simulink model "SIM_PEM_stack"  (R2020b)
settings: Solver=VariableStepAuto  StartTime=0.0  StopTime=60e3  RelTol=1e-3
undefined symbols (not defined in the file or in its folder): FC, FuelCellLoadFcn, gcbh, sps_rtmsupport
libraries: powerlib x106, simulink x22, spsFuelCellModel x21, dspswit3 x1, mylib x1
(part 3 of 3)

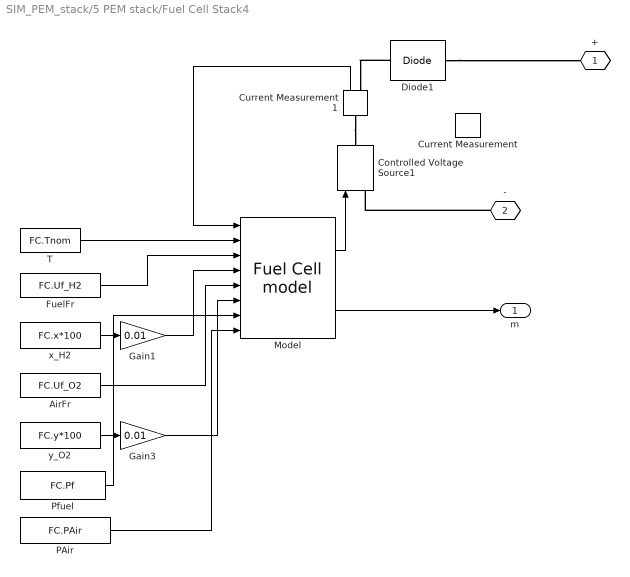
== system SIM_PEM_stack/5 PEM stack/Fuel Cell Stack4 ==
  AirFr : Constant  Value=FC.Uf_O2
  Controlled Voltage Source1 : powerlib/Electrical Sources/Controlled Voltage Source  Initialize=on  Source_Type=AC  Amplitude=0  Phase=0  Frequency=0  Measurements=None
  Current Measurement : powerlib/Measurements/Current Measurement  PhasorSimulation=off  OutputType=Complex  PSBequivalent=0
  Current Measurement1 : powerlib/Measurements/Current Measurement  PhasorSimulation=off  OutputType=Complex  PSBequivalent=0
  Diode1 : powerlib/Power Electronics/Diode  Ron=FC.Rohm  Lon=0  Vf=0  IC=0  UseSnubber=off  Rs=1e4  Cs=inf  Measurements=off
  FuelFr : Constant  Value=FC.Uf_H2
  Gain1 : Gain  Gain=0.01
  Gain3 : Gain  Gain=0.01
  Model : spsFuelCellModel/Fuel Cell model  SystemSampleTime=-1  LabelModeActiveChoice=Continuous/Detailed  VariantActivationTime=update diagram  Latency=0  AutoFrameSizeCalculation=off
      settings: AttributesFormatString=%<BlockChoice>  SourceProductBaseCode=PS
  PAir : Constant  Value=FC.PAir
  Pfuel : Constant  Value=FC.Pf
  T : Constant  Value=FC.Tnom
  x_H2 : Constant  Value=FC.x*100
  y_O2 : Constant  Value=FC.y*100
  + : PMIOPort  Tag=PMCPort  Side=Right
  - : PMIOPort  Tag=PMCPort  Port=2  Side=Right
  m : Outport  VectorParamsAs1DForOutWhenUnconnected=off
  wires:
  PAir/1 -> Model/8
  Pfuel/1 -> Model/7
  T/1 -> Model/2
  Model/1 -> Controlled Voltage Source1/1
  Current Measurement1/1 -> Model/1
  Model/2 -> m/1
  FuelFr/1 -> Model/3
  x_H2/1 -> Gain1/1
  AirFr/1 -> Model/5
  y_O2/1 -> Gain3/1
  Gain1/1 -> Model/4
  Gain3/1 -> Model/6
  connections:
  Current Measurement1/LConn1 -- Controlled Voltage Source1/RConn1
  Diode1/LConn1 -- Current Measurement1/RConn1
  -/RConn1 -- Controlled Voltage Source1/LConn1
  Diode1/RConn1 -- +/RConn1

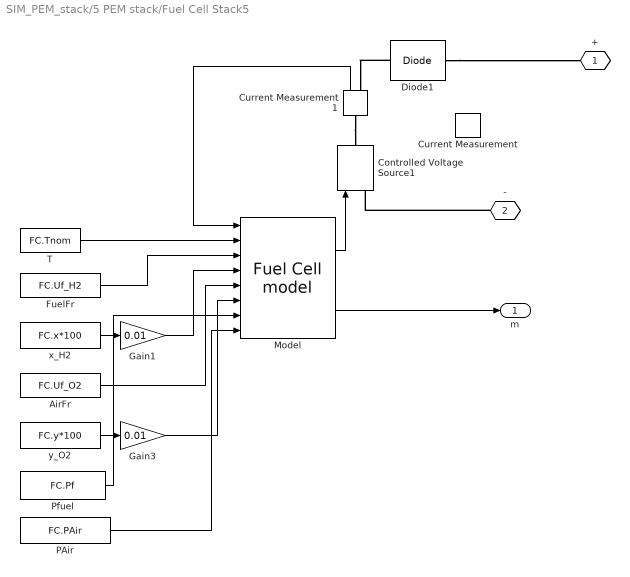
== system SIM_PEM_stack/5 PEM stack/Fuel Cell Stack5 ==
  AirFr : Constant  Value=FC.Uf_O2
  Controlled Voltage Source1 : powerlib/Electrical Sources/Controlled Voltage Source  Initialize=on  Source_Type=AC  Amplitude=0  Phase=0  Frequency=0  Measurements=None
  Current Measurement : powerlib/Measurements/Current Measurement  PhasorSimulation=off  OutputType=Complex  PSBequivalent=0
  Current Measurement1 : powerlib/Measurements/Current Measurement  PhasorSimulation=off  OutputType=Complex  PSBequivalent=0
  Diode1 : powerlib/Power Electronics/Diode  Ron=FC.Rohm  Lon=0  Vf=0  IC=0  UseSnubber=off  Rs=1e4  Cs=inf  Measurements=off
  FuelFr : Constant  Value=FC.Uf_H2
  Gain1 : Gain  Gain=0.01
  Gain3 : Gain  Gain=0.01
  Model : spsFuelCellModel/Fuel Cell model  SystemSampleTime=-1  LabelModeActiveChoice=Continuous/Detailed  VariantActivationTime=update diagram  Latency=0  AutoFrameSizeCalculation=off
      settings: AttributesFormatString=%<BlockChoice>  SourceProductBaseCode=PS
  PAir : Constant  Value=FC.PAir
  Pfuel : Constant  Value=FC.Pf
  T : Constant  Value=FC.Tnom
  x_H2 : Constant  Value=FC.x*100
  y_O2 : Constant  Value=FC.y*100
  + : PMIOPort  Tag=PMCPort  Side=Right
  - : PMIOPort  Tag=PMCPort  Port=2  Side=Right
  m : Outport  VectorParamsAs1DForOutWhenUnconnected=off
  wires:
  PAir/1 -> Model/8
  Pfuel/1 -> Model/7
  T/1 -> Model/2
  Model/1 -> Controlled Voltage Source1/1
  Current Measurement1/1 -> Model/1
  Model/2 -> m/1
  FuelFr/1 -> Model/3
  x_H2/1 -> Gain1/1
  AirFr/1 -> Model/5
  y_O2/1 -> Gain3/1
  Gain1/1 -> Model/4
  Gain3/1 -> Model/6
  connections:
  Current Measurement1/LConn1 -- Controlled Voltage Source1/RConn1
  Diode1/LConn1 -- Current Measurement1/RConn1
  -/RConn1 -- Controlled Voltage Source1/LConn1
  Diode1/RConn1 -- +/RConn1

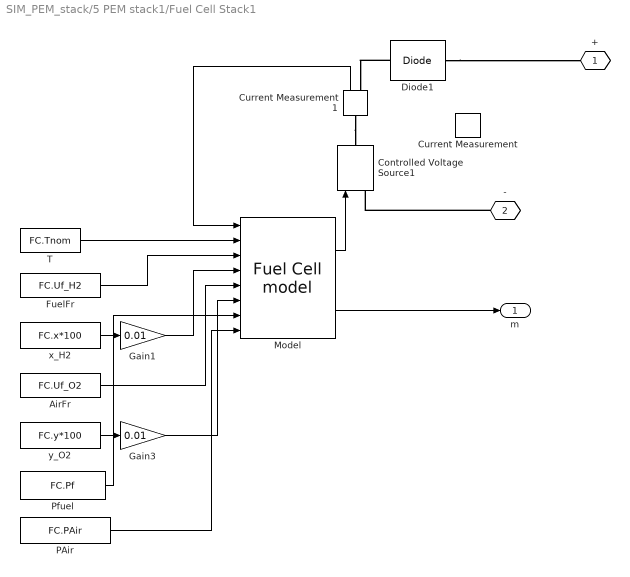
== system SIM_PEM_stack/5 PEM stack1/Fuel Cell Stack1 ==
  AirFr : Constant  Value=FC.Uf_O2
  Controlled Voltage Source1 : powerlib/Electrical Sources/Controlled Voltage Source  Initialize=on  Source_Type=AC  Amplitude=0  Phase=0  Frequency=0  Measurements=None
  Current Measurement : powerlib/Measurements/Current Measurement  PhasorSimulation=off  OutputType=Complex  PSBequivalent=0
  Current Measurement1 : powerlib/Measurements/Current Measurement  PhasorSimulation=off  OutputType=Complex  PSBequivalent=0
  Diode1 : powerlib/Power Electronics/Diode  Ron=FC.Rohm  Lon=0  Vf=0  IC=0  UseSnubber=off  Rs=1e4  Cs=inf  Measurements=off
  FuelFr : Constant  Value=FC.Uf_H2
  Gain1 : Gain  Gain=0.01
  Gain3 : Gain  Gain=0.01
  Model : spsFuelCellModel/Fuel Cell model  SystemSampleTime=-1  LabelModeActiveChoice=Continuous/Detailed  VariantActivationTime=update diagram  Latency=0  AutoFrameSizeCalculation=off
      settings: AttributesFormatString=%<BlockChoice>  SourceProductBaseCode=PS
  PAir : Constant  Value=FC.PAir
  Pfuel : Constant  Value=FC.Pf
  T : Constant  Value=FC.Tnom
  x_H2 : Constant  Value=FC.x*100
  y_O2 : Constant  Value=FC.y*100
  + : PMIOPort  Tag=PMCPort  Side=Right
  - : PMIOPort  Tag=PMCPort  Port=2  Side=Right
  m : Outport  VectorParamsAs1DForOutWhenUnconnected=off
  wires:
  PAir/1 -> Model/8
  Pfuel/1 -> Model/7
  T/1 -> Model/2
  Model/1 -> Controlled Voltage Source1/1
  Current Measurement1/1 -> Model/1
  Model/2 -> m/1
  FuelFr/1 -> Model/3
  x_H2/1 -> Gain1/1
  AirFr/1 -> Model/5
  y_O2/1 -> Gain3/1
  Gain1/1 -> Model/4
  Gain3/1 -> Model/6
  connections:
  Current Measurement1/LConn1 -- Controlled Voltage Source1/RConn1
  Diode1/LConn1 -- Current Measurement1/RConn1
  -/RConn1 -- Controlled Voltage Source1/LConn1
  Diode1/RConn1 -- +/RConn1

== system SIM_PEM_stack/5 PEM stack1/Fuel Cell Stack2 ==
  AirFr : Constant  Value=FC.Uf_O2
  Controlled Voltage Source1 : powerlib/Electrical Sources/Controlled Voltage Source  Initialize=on  Source_Type=AC  Amplitude=0  Phase=0  Frequency=0  Measurements=None
  Current Measurement : powerlib/Measurements/Current Measurement  PhasorSimulation=off  OutputType=Complex  PSBequivalent=0
  Current Measurement1 : powerlib/Measurements/Current Measurement  PhasorSimulation=off  OutputType=Complex  PSBequivalent=0
  Diode1 : powerlib/Power Electronics/Diode  Ron=FC.Rohm  Lon=0  Vf=0  IC=0  UseSnubber=off  Rs=1e4  Cs=inf  Measurements=off
  FuelFr : Constant  Value=FC.Uf_H2
  Gain1 : Gain  Gain=0.01
  Gain3 : Gain  Gain=0.01
  Model : spsFuelCellModel/Fuel Cell model  SystemSampleTime=-1  LabelModeActiveChoice=Continuous/Detailed  VariantActivationTime=update diagram  Latency=0  AutoFrameSizeCalculation=off
      settings: AttributesFormatString=%<BlockChoice>  SourceProductBaseCode=PS
  PAir : Constant  Value=FC.PAir
  Pfuel : Constant  Value=FC.Pf
  T : Constant  Value=FC.Tnom
  x_H2 : Constant  Value=FC.x*100
  y_O2 : Constant  Value=FC.y*100
  + : PMIOPort  Tag=PMCPort  Side=Right
  - : PMIOPort  Tag=PMCPort  Port=2  Side=Right
  m : Outport  VectorParamsAs1DForOutWhenUnconnected=off
  wires:
  PAir/1 -> Model/8
  Pfuel/1 -> Model/7
  T/1 -> Model/2
  Model/1 -> Controlled Voltage Source1/1
  Current Measurement1/1 -> Model/1
  Model/2 -> m/1
  FuelFr/1 -> Model/3
  x_H2/1 -> Gain1/1
  AirFr/1 -> Model/5
  y_O2/1 -> Gain3/1
  Gain1/1 -> Model/4
  Gain3/1 -> Model/6
  connections:
  Current Measurement1/LConn1 -- Controlled Voltage Source1/RConn1
  Diode1/LConn1 -- Current Measurement1/RConn1
  -/RConn1 -- Controlled Voltage Source1/LConn1
  Diode1/RConn1 -- +/RConn1

== system SIM_PEM_stack/5 PEM stack1/Fuel Cell Stack3 ==
  AirFr : Constant  Value=FC.Uf_O2
  Controlled Voltage Source1 : powerlib/Electrical Sources/Controlled Voltage Source  Initialize=on  Source_Type=AC  Amplitude=0  Phase=0  Frequency=0  Measurements=None
  Current Measurement : powerlib/Measurements/Current Measurement  PhasorSimulation=off  OutputType=Complex  PSBequivalent=0
  Current Measurement1 : powerlib/Measurements/Current Measurement  PhasorSimulation=off  OutputType=Complex  PSBequivalent=0
  Diode1 : powerlib/Power Electronics/Diode  Ron=FC.Rohm  Lon=0  Vf=0  IC=0  UseSnubber=off  Rs=1e4  Cs=inf  Measurements=off
  FuelFr : Constant  Value=FC.Uf_H2
  Gain1 : Gain  Gain=0.01
  Gain3 : Gain  Gain=0.01
  Model : spsFuelCellModel/Fuel Cell model  SystemSampleTime=-1  LabelModeActiveChoice=Continuous/Detailed  VariantActivationTime=update diagram  Latency=0  AutoFrameSizeCalculation=off
      settings: AttributesFormatString=%<BlockChoice>  SourceProductBaseCode=PS
  PAir : Constant  Value=FC.PAir
  Pfuel : Constant  Value=FC.Pf
  T : Constant  Value=FC.Tnom
  x_H2 : Constant  Value=FC.x*100
  y_O2 : Constant  Value=FC.y*100
  + : PMIOPort  Tag=PMCPort  Side=Right
  - : PMIOPort  Tag=PMCPort  Port=2  Side=Right
  m : Outport  VectorParamsAs1DForOutWhenUnconnected=off
  wires:
  PAir/1 -> Model/8
  Pfuel/1 -> Model/7
  T/1 -> Model/2
  Model/1 -> Controlled Voltage Source1/1
  Current Measurement1/1 -> Model/1
  Model/2 -> m/1
  FuelFr/1 -> Model/3
  x_H2/1 -> Gain1/1
  AirFr/1 -> Model/5
  y_O2/1 -> Gain3/1
  Gain1/1 -> Model/4
  Gain3/1 -> Model/6
  connections:
  Current Measurement1/LConn1 -- Controlled Voltage Source1/RConn1
  Diode1/LConn1 -- Current Measurement1/RConn1
  -/RConn1 -- Controlled Voltage Source1/LConn1
  Diode1/RConn1 -- +/RConn1

== system SIM_PEM_stack/5 PEM stack1/Fuel Cell Stack4 ==
  AirFr : Constant  Value=FC.Uf_O2
  Controlled Voltage Source1 : powerlib/Electrical Sources/Controlled Voltage Source  Initialize=on  Source_Type=AC  Amplitude=0  Phase=0  Frequency=0  Measurements=None
  Current Measurement : powerlib/Measurements/Current Measurement  PhasorSimulation=off  OutputType=Complex  PSBequivalent=0
  Current Measurement1 : powerlib/Measurements/Current Measurement  PhasorSimulation=off  OutputType=Complex  PSBequivalent=0
  Diode1 : powerlib/Power Electronics/Diode  Ron=FC.Rohm  Lon=0  Vf=0  IC=0  UseSnubber=off  Rs=1e4  Cs=inf  Measurements=off
  FuelFr : Constant  Value=FC.Uf_H2
  Gain1 : Gain  Gain=0.01
  Gain3 : Gain  Gain=0.01
  Model : spsFuelCellModel/Fuel Cell model  SystemSampleTime=-1  LabelModeActiveChoice=Continuous/Detailed  VariantActivationTime=update diagram  Latency=0  AutoFrameSizeCalculation=off
      settings: AttributesFormatString=%<BlockChoice>  SourceProductBaseCode=PS
  PAir : Constant  Value=FC.PAir
  Pfuel : Constant  Value=FC.Pf
  T : Constant  Value=FC.Tnom
  x_H2 : Constant  Value=FC.x*100
  y_O2 : Constant  Value=FC.y*100
  + : PMIOPort  Tag=PMCPort  Side=Right
  - : PMIOPort  Tag=PMCPort  Port=2  Side=Right
  m : Outport  VectorParamsAs1DForOutWhenUnconnected=off
  wires:
  PAir/1 -> Model/8
  Pfuel/1 -> Model/7
  T/1 -> Model/2
  Model/1 -> Controlled Voltage Source1/1
  Current Measurement1/1 -> Model/1
  Model/2 -> m/1
  FuelFr/1 -> Model/3
  x_H2/1 -> Gain1/1
  AirFr/1 -> Model/5
  y_O2/1 -> Gain3/1
  Gain1/1 -> Model/4
  Gain3/1 -> Model/6
  connections:
  Current Measurement1/LConn1 -- Controlled Voltage Source1/RConn1
  Diode1/LConn1 -- Current Measurement1/RConn1
  -/RConn1 -- Controlled Voltage Source1/LConn1
  Diode1/RConn1 -- +/RConn1

== system SIM_PEM_stack/5 PEM stack1/Fuel Cell Stack5 ==
  AirFr : Constant  Value=FC.Uf_O2
  Controlled Voltage Source1 : powerlib/Electrical Sources/Controlled Voltage Source  Initialize=on  Source_Type=AC  Amplitude=0  Phase=0  Frequency=0  Measurements=None
  Current Measurement : powerlib/Measurements/Current Measurement  PhasorSimulation=off  OutputType=Complex  PSBequivalent=0
  Current Measurement1 : powerlib/Measurements/Current Measurement  PhasorSimulation=off  OutputType=Complex  PSBequivalent=0
  Diode1 : powerlib/Power Electronics/Diode  Ron=FC.Rohm  Lon=0  Vf=0  IC=0  UseSnubber=off  Rs=1e4  Cs=inf  Measurements=off
  FuelFr : Constant  Value=FC.Uf_H2
  Gain1 : Gain  Gain=0.01
  Gain3 : Gain  Gain=0.01
  Model : spsFuelCellModel/Fuel Cell model  SystemSampleTime=-1  LabelModeActiveChoice=Continuous/Detailed  VariantActivationTime=update diagram  Latency=0  AutoFrameSizeCalculation=off
      settings: AttributesFormatString=%<BlockChoice>  SourceProductBaseCode=PS
  PAir : Constant  Value=FC.PAir
  Pfuel : Constant  Value=FC.Pf
  T : Constant  Value=FC.Tnom
  x_H2 : Constant  Value=FC.x*100
  y_O2 : Constant  Value=FC.y*100
  + : PMIOPort  Tag=PMCPort  Side=Right
  - : PMIOPort  Tag=PMCPort  Port=2  Side=Right
  m : Outport  VectorParamsAs1DForOutWhenUnconnected=off
  wires:
  PAir/1 -> Model/8
  Pfuel/1 -> Model/7
  T/1 -> Model/2
  Model/1 -> Controlled Voltage Source1/1
  Current Measurement1/1 -> Model/1
  Model/2 -> m/1
  FuelFr/1 -> Model/3
  x_H2/1 -> Gain1/1
  AirFr/1 -> Model/5
  y_O2/1 -> Gain3/1
  Gain1/1 -> Model/4
  Gain3/1 -> Model/6
  connections:
  Current Measurement1/LConn1 -- Controlled Voltage Source1/RConn1
  Diode1/LConn1 -- Current Measurement1/RConn1
  -/RConn1 -- Controlled Voltage Source1/LConn1
  Diode1/RConn1 -- +/RConn1

== system SIM_PEM_stack/5 PEM stack2/Fuel Cell Stack1 ==
  AirFr : Constant  Value=FC.Uf_O2
  Controlled Voltage Source1 : powerlib/Electrical Sources/Controlled Voltage Source  Initialize=on  Source_Type=AC  Amplitude=0  Phase=0  Frequency=0  Measurements=None
  Current Measurement : powerlib/Measurements/Current Measurement  PhasorSimulation=off  OutputType=Complex  PSBequivalent=0
  Current Measurement1 : powerlib/Measurements/Current Measurement  PhasorSimulation=off  OutputType=Complex  PSBequivalent=0
  Diode1 : powerlib/Power Electronics/Diode  Ron=FC.Rohm  Lon=0  Vf=0  IC=0  UseSnubber=off  Rs=1e4  Cs=inf  Measurements=off
  FuelFr : Constant  Value=FC.Uf_H2
  Gain1 : Gain  Gain=0.01
  Gain3 : Gain  Gain=0.01
  Model : spsFuelCellModel/Fuel Cell model  SystemSampleTime=-1  LabelModeActiveChoice=Continuous/Detailed  VariantActivationTime=update diagram  Latency=0  AutoFrameSizeCalculation=off
      settings: AttributesFormatString=%<BlockChoice>  SourceProductBaseCode=PS
  PAir : Constant  Value=FC.PAir
  Pfuel : Constant  Value=FC.Pf
  T : Constant  Value=FC.Tnom
  x_H2 : Constant  Value=FC.x*100
  y_O2 : Constant  Value=FC.y*100
  + : PMIOPort  Tag=PMCPort  Side=Right
  - : PMIOPort  Tag=PMCPort  Port=2  Side=Right
  m : Outport  VectorParamsAs1DForOutWhenUnconnected=off
  wires:
  PAir/1 -> Model/8
  Pfuel/1 -> Model/7
  T/1 -> Model/2
  Model/1 -> Controlled Voltage Source1/1
  Current Measurement1/1 -> Model/1
  Model/2 -> m/1
  FuelFr/1 -> Model/3
  x_H2/1 -> Gain1/1
  AirFr/1 -> Model/5
  y_O2/1 -> Gain3/1
  Gain1/1 -> Model/4
  Gain3/1 -> Model/6
  connections:
  Current Measurement1/LConn1 -- Controlled Voltage Source1/RConn1
  Diode1/LConn1 -- Current Measurement1/RConn1
  -/RConn1 -- Controlled Voltage Source1/LConn1
  Diode1/RConn1 -- +/RConn1

== system SIM_PEM_stack/5 PEM stack2/Fuel Cell Stack2 ==
  AirFr : Constant  Value=FC.Uf_O2
  Controlled Voltage Source1 : powerlib/Electrical Sources/Controlled Voltage Source  Initialize=on  Source_Type=AC  Amplitude=0  Phase=0  Frequency=0  Measurements=None
  Current Measurement : powerlib/Measurements/Current Measurement  PhasorSimulation=off  OutputType=Complex  PSBequivalent=0
  Current Measurement1 : powerlib/Measurements/Current Measurement  PhasorSimulation=off  OutputType=Complex  PSBequivalent=0
  Diode1 : powerlib/Power Electronics/Diode  Ron=FC.Rohm  Lon=0  Vf=0  IC=0  UseSnubber=off  Rs=1e4  Cs=inf  Measurements=off
  FuelFr : Constant  Value=FC.Uf_H2
  Gain1 : Gain  Gain=0.01
  Gain3 : Gain  Gain=0.01
  Model : spsFuelCellModel/Fuel Cell model  SystemSampleTime=-1  LabelModeActiveChoice=Continuous/Detailed  VariantActivationTime=update diagram  Latency=0  AutoFrameSizeCalculation=off
      settings: AttributesFormatString=%<BlockChoice>  SourceProductBaseCode=PS
  PAir : Constant  Value=FC.PAir
  Pfuel : Constant  Value=FC.Pf
  T : Constant  Value=FC.Tnom
  x_H2 : Constant  Value=FC.x*100
  y_O2 : Constant  Value=FC.y*100
  + : PMIOPort  Tag=PMCPort  Side=Right
  - : PMIOPort  Tag=PMCPort  Port=2  Side=Right
  m : Outport  VectorParamsAs1DForOutWhenUnconnected=off
  wires:
  PAir/1 -> Model/8
  Pfuel/1 -> Model/7
  T/1 -> Model/2
  Model/1 -> Controlled Voltage Source1/1
  Current Measurement1/1 -> Model/1
  Model/2 -> m/1
  FuelFr/1 -> Model/3
  x_H2/1 -> Gain1/1
  AirFr/1 -> Model/5
  y_O2/1 -> Gain3/1
  Gain1/1 -> Model/4
  Gain3/1 -> Model/6
  connections:
  Current Measurement1/LConn1 -- Controlled Voltage Source1/RConn1
  Diode1/LConn1 -- Current Measurement1/RConn1
  -/RConn1 -- Controlled Voltage Source1/LConn1
  Diode1/RConn1 -- +/RConn1

== system SIM_PEM_stack/5 PEM stack2/Fuel Cell Stack3 ==
  AirFr : Constant  Value=FC.Uf_O2
  Controlled Voltage Source1 : powerlib/Electrical Sources/Controlled Voltage Source  Initialize=on  Source_Type=AC  Amplitude=0  Phase=0  Frequency=0  Measurements=None
  Current Measurement : powerlib/Measurements/Current Measurement  PhasorSimulation=off  OutputType=Complex  PSBequivalent=0
  Current Measurement1 : powerlib/Measurements/Current Measurement  PhasorSimulation=off  OutputType=Complex  PSBequivalent=0
  Diode1 : powerlib/Power Electronics/Diode  Ron=FC.Rohm  Lon=0  Vf=0  IC=0  UseSnubber=off  Rs=1e4  Cs=inf  Measurements=off
  FuelFr : Constant  Value=FC.Uf_H2
  Gain1 : Gain  Gain=0.01
  Gain3 : Gain  Gain=0.01
  Model : spsFuelCellModel/Fuel Cell model  SystemSampleTime=-1  LabelModeActiveChoice=Continuous/Detailed  VariantActivationTime=update diagram  Latency=0  AutoFrameSizeCalculation=off
      settings: AttributesFormatString=%<BlockChoice>  SourceProductBaseCode=PS
  PAir : Constant  Value=FC.PAir
  Pfuel : Constant  Value=FC.Pf
  T : Constant  Value=FC.Tnom
  x_H2 : Constant  Value=FC.x*100
  y_O2 : Constant  Value=FC.y*100
  + : PMIOPort  Tag=PMCPort  Side=Right
  - : PMIOPort  Tag=PMCPort  Port=2  Side=Right
  m : Outport  VectorParamsAs1DForOutWhenUnconnected=off
  wires:
  PAir/1 -> Model/8
  Pfuel/1 -> Model/7
  T/1 -> Model/2
  Model/1 -> Controlled Voltage Source1/1
  Current Measurement1/1 -> Model/1
  Model/2 -> m/1
  FuelFr/1 -> Model/3
  x_H2/1 -> Gain1/1
  AirFr/1 -> Model/5
  y_O2/1 -> Gain3/1
  Gain1/1 -> Model/4
  Gain3/1 -> Model/6
  connections:
  Current Measurement1/LConn1 -- Controlled Voltage Source1/RConn1
  Diode1/LConn1 -- Current Measurement1/RConn1
  -/RConn1 -- Controlled Voltage Source1/LConn1
  Diode1/RConn1 -- +/RConn1

== system SIM_PEM_stack/5 PEM stack2/Fuel Cell Stack4 ==
  AirFr : Constant  Value=FC.Uf_O2
  Controlled Voltage Source1 : powerlib/Electrical Sources/Controlled Voltage Source  Initialize=on  Source_Type=AC  Amplitude=0  Phase=0  Frequency=0  Measurements=None
  Current Measurement : powerlib/Measurements/Current Measurement  PhasorSimulation=off  OutputType=Complex  PSBequivalent=0
  Current Measurement1 : powerlib/Measurements/Current Measurement  PhasorSimulation=off  OutputType=Complex  PSBequivalent=0
  Diode1 : powerlib/Power Electronics/Diode  Ron=FC.Rohm  Lon=0  Vf=0  IC=0  UseSnubber=off  Rs=1e4  Cs=inf  Measurements=off
  FuelFr : Constant  Value=FC.Uf_H2
  Gain1 : Gain  Gain=0.01
  Gain3 : Gain  Gain=0.01
  Model : spsFuelCellModel/Fuel Cell model  SystemSampleTime=-1  LabelModeActiveChoice=Continuous/Detailed  VariantActivationTime=update diagram  Latency=0  AutoFrameSizeCalculation=off
      settings: AttributesFormatString=%<BlockChoice>  SourceProductBaseCode=PS
  PAir : Constant  Value=FC.PAir
  Pfuel : Constant  Value=FC.Pf
  T : Constant  Value=FC.Tnom
  x_H2 : Constant  Value=FC.x*100
  y_O2 : Constant  Value=FC.y*100
  + : PMIOPort  Tag=PMCPort  Side=Right
  - : PMIOPort  Tag=PMCPort  Port=2  Side=Right
  m : Outport  VectorParamsAs1DForOutWhenUnconnected=off
  wires:
  PAir/1 -> Model/8
  Pfuel/1 -> Model/7
  T/1 -> Model/2
  Model/1 -> Controlled Voltage Source1/1
  Current Measurement1/1 -> Model/1
  Model/2 -> m/1
  FuelFr/1 -> Model/3
  x_H2/1 -> Gain1/1
  AirFr/1 -> Model/5
  y_O2/1 -> Gain3/1
  Gain1/1 -> Model/4
  Gain3/1 -> Model/6
  connections:
  Current Measurement1/LConn1 -- Controlled Voltage Source1/RConn1
  Diode1/LConn1 -- Current Measurement1/RConn1
  -/RConn1 -- Controlled Voltage Source1/LConn1
  Diode1/RConn1 -- +/RConn1

== system SIM_PEM_stack/5 PEM stack2/Fuel Cell Stack5 ==
  AirFr : Constant  Value=FC.Uf_O2
  Controlled Voltage Source1 : powerlib/Electrical Sources/Controlled Voltage Source  Initialize=on  Source_Type=AC  Amplitude=0  Phase=0  Frequency=0  Measurements=None
  Current Measurement : powerlib/Measurements/Current Measurement  PhasorSimulation=off  OutputType=Complex  PSBequivalent=0
  Current Measurement1 : powerlib/Measurements/Current Measurement  PhasorSimulation=off  OutputType=Complex  PSBequivalent=0
  Diode1 : powerlib/Power Electronics/Diode  Ron=FC.Rohm  Lon=0  Vf=0  IC=0  UseSnubber=off  Rs=1e4  Cs=inf  Measurements=off
  FuelFr : Constant  Value=FC.Uf_H2
  Gain1 : Gain  Gain=0.01
  Gain3 : Gain  Gain=0.01
  Model : spsFuelCellModel/Fuel Cell model  SystemSampleTime=-1  LabelModeActiveChoice=Continuous/Detailed  VariantActivationTime=update diagram  Latency=0  AutoFrameSizeCalculation=off
      settings: AttributesFormatString=%<BlockChoice>  SourceProductBaseCode=PS
  PAir : Constant  Value=FC.PAir
  Pfuel : Constant  Value=FC.Pf
  T : Constant  Value=FC.Tnom
  x_H2 : Constant  Value=FC.x*100
  y_O2 : Constant  Value=FC.y*100
  + : PMIOPort  Tag=PMCPort  Side=Right
  - : PMIOPort  Tag=PMCPort  Port=2  Side=Right
  m : Outport  VectorParamsAs1DForOutWhenUnconnected=off
  wires:
  PAir/1 -> Model/8
  Pfuel/1 -> Model/7
  T/1 -> Model/2
  Model/1 -> Controlled Voltage Source1/1
  Current Measurement1/1 -> Model/1
  Model/2 -> m/1
  FuelFr/1 -> Model/3
  x_H2/1 -> Gain1/1
  AirFr/1 -> Model/5
  y_O2/1 -> Gain3/1
  Gain1/1 -> Model/4
  Gain3/1 -> Model/6
  connections:
  Current Measurement1/LConn1 -- Controlled Voltage Source1/RConn1
  Diode1/LConn1 -- Current Measurement1/RConn1
  -/RConn1 -- Controlled Voltage Source1/LConn1
  Diode1/RConn1 -- +/RConn1

== system SIM_PEM_stack/5 PEM stack3/Fuel Cell Stack1 ==
  AirFr : Constant  Value=FC.Uf_O2
  Controlled Voltage Source1 : powerlib/Electrical Sources/Controlled Voltage Source  Initialize=on  Source_Type=AC  Amplitude=0  Phase=0  Frequency=0  Measurements=None
  Current Measurement : powerlib/Measurements/Current Measurement  PhasorSimulation=off  OutputType=Complex  PSBequivalent=0
  Current Measurement1 : powerlib/Measurements/Current Measurement  PhasorSimulation=off  OutputType=Complex  PSBequivalent=0
  Diode1 : powerlib/Power Electronics/Diode  Ron=FC.Rohm  Lon=0  Vf=0  IC=0  UseSnubber=off  Rs=1e4  Cs=inf  Measurements=off
  FuelFr : Constant  Value=FC.Uf_H2
  Gain1 : Gain  Gain=0.01
  Gain3 : Gain  Gain=0.01
  Model : spsFuelCellModel/Fuel Cell model  SystemSampleTime=-1  LabelModeActiveChoice=Continuous/Detailed  VariantActivationTime=update diagram  Latency=0  AutoFrameSizeCalculation=off
      settings: AttributesFormatString=%<BlockChoice>  SourceProductBaseCode=PS
  PAir : Constant  Value=FC.PAir
  Pfuel : Constant  Value=FC.Pf
  T : Constant  Value=FC.Tnom
  x_H2 : Constant  Value=FC.x*100
  y_O2 : Constant  Value=FC.y*100
  + : PMIOPort  Tag=PMCPort  Side=Right
  - : PMIOPort  Tag=PMCPort  Port=2  Side=Right
  m : Outport  VectorParamsAs1DForOutWhenUnconnected=off
  wires:
  PAir/1 -> Model/8
  Pfuel/1 -> Model/7
  T/1 -> Model/2
  Model/1 -> Controlled Voltage Source1/1
  Current Measurement1/1 -> Model/1
  Model/2 -> m/1
  FuelFr/1 -> Model/3
  x_H2/1 -> Gain1/1
  AirFr/1 -> Model/5
  y_O2/1 -> Gain3/1
  Gain1/1 -> Model/4
  Gain3/1 -> Model/6
  connections:
  Current Measurement1/LConn1 -- Controlled Voltage Source1/RConn1
  Diode1/LConn1 -- Current Measurement1/RConn1
  -/RConn1 -- Controlled Voltage Source1/LConn1
  Diode1/RConn1 -- +/RConn1

== system SIM_PEM_stack/5 PEM stack3/Fuel Cell Stack2 ==
  AirFr : Constant  Value=FC.Uf_O2
  Controlled Voltage Source1 : powerlib/Electrical Sources/Controlled Voltage Source  Initialize=on  Source_Type=AC  Amplitude=0  Phase=0  Frequency=0  Measurements=None
  Current Measurement : powerlib/Measurements/Current Measurement  PhasorSimulation=off  OutputType=Complex  PSBequivalent=0
  Current Measurement1 : powerlib/Measurements/Current Measurement  PhasorSimulation=off  OutputType=Complex  PSBequivalent=0
  Diode1 : powerlib/Power Electronics/Diode  Ron=FC.Rohm  Lon=0  Vf=0  IC=0  UseSnubber=off  Rs=1e4  Cs=inf  Measurements=off
  FuelFr : Constant  Value=FC.Uf_H2
  Gain1 : Gain  Gain=0.01
  Gain3 : Gain  Gain=0.01
  Model : spsFuelCellModel/Fuel Cell model  SystemSampleTime=-1  LabelModeActiveChoice=Continuous/Detailed  VariantActivationTime=update diagram  Latency=0  AutoFrameSizeCalculation=off
      settings: AttributesFormatString=%<BlockChoice>  SourceProductBaseCode=PS
  PAir : Constant  Value=FC.PAir
  Pfuel : Constant  Value=FC.Pf
  T : Constant  Value=FC.Tnom
  x_H2 : Constant  Value=FC.x*100
  y_O2 : Constant  Value=FC.y*100
  + : PMIOPort  Tag=PMCPort  Side=Right
  - : PMIOPort  Tag=PMCPort  Port=2  Side=Right
  m : Outport  VectorParamsAs1DForOutWhenUnconnected=off
  wires:
  PAir/1 -> Model/8
  Pfuel/1 -> Model/7
  T/1 -> Model/2
  Model/1 -> Controlled Voltage Source1/1
  Current Measurement1/1 -> Model/1
  Model/2 -> m/1
  FuelFr/1 -> Model/3
  x_H2/1 -> Gain1/1
  AirFr/1 -> Model/5
  y_O2/1 -> Gain3/1
  Gain1/1 -> Model/4
  Gain3/1 -> Model/6
  connections:
  Current Measurement1/LConn1 -- Controlled Voltage Source1/RConn1
  Diode1/LConn1 -- Current Measurement1/RConn1
  -/RConn1 -- Controlled Voltage Source1/LConn1
  Diode1/RConn1 -- +/RConn1

== system SIM_PEM_stack/5 PEM stack3/Fuel Cell Stack3 ==
  AirFr : Constant  Value=FC.Uf_O2
  Controlled Voltage Source1 : powerlib/Electrical Sources/Controlled Voltage Source  Initialize=on  Source_Type=AC  Amplitude=0  Phase=0  Frequency=0  Measurements=None
  Current Measurement : powerlib/Measurements/Current Measurement  PhasorSimulation=off  OutputType=Complex  PSBequivalent=0
  Current Measurement1 : powerlib/Measurements/Current Measurement  PhasorSimulation=off  OutputType=Complex  PSBequivalent=0
  Diode1 : powerlib/Power Electronics/Diode  Ron=FC.Rohm  Lon=0  Vf=0  IC=0  UseSnubber=off  Rs=1e4  Cs=inf  Measurements=off
  FuelFr : Constant  Value=FC.Uf_H2
  Gain1 : Gain  Gain=0.01
  Gain3 : Gain  Gain=0.01
  Model : spsFuelCellModel/Fuel Cell model  SystemSampleTime=-1  LabelModeActiveChoice=Continuous/Detailed  VariantActivationTime=update diagram  Latency=0  AutoFrameSizeCalculation=off
      settings: AttributesFormatString=%<BlockChoice>  SourceProductBaseCode=PS
  PAir : Constant  Value=FC.PAir
  Pfuel : Constant  Value=FC.Pf
  T : Constant  Value=FC.Tnom
  x_H2 : Constant  Value=FC.x*100
  y_O2 : Constant  Value=FC.y*100
  + : PMIOPort  Tag=PMCPort  Side=Right
  - : PMIOPort  Tag=PMCPort  Port=2  Side=Right
  m : Outport  VectorParamsAs1DForOutWhenUnconnected=off
  wires:
  PAir/1 -> Model/8
  Pfuel/1 -> Model/7
  T/1 -> Model/2
  Model/1 -> Controlled Voltage Source1/1
  Current Measurement1/1 -> Model/1
  Model/2 -> m/1
  FuelFr/1 -> Model/3
  x_H2/1 -> Gain1/1
  AirFr/1 -> Model/5
  y_O2/1 -> Gain3/1
  Gain1/1 -> Model/4
  Gain3/1 -> Model/6
  connections:
  Current Measurement1/LConn1 -- Controlled Voltage Source1/RConn1
  Diode1/LConn1 -- Current Measurement1/RConn1
  -/RConn1 -- Controlled Voltage Source1/LConn1
  Diode1/RConn1 -- +/RConn1

== system SIM_PEM_stack/5 PEM stack3/Fuel Cell Stack4 ==
  AirFr : Constant  Value=FC.Uf_O2
  Controlled Voltage Source1 : powerlib/Electrical Sources/Controlled Voltage Source  Initialize=on  Source_Type=AC  Amplitude=0  Phase=0  Frequency=0  Measurements=None
  Current Measurement : powerlib/Measurements/Current Measurement  PhasorSimulation=off  OutputType=Complex  PSBequivalent=0
  Current Measurement1 : powerlib/Measurements/Current Measurement  PhasorSimulation=off  OutputType=Complex  PSBequivalent=0
  Diode1 : powerlib/Power Electronics/Diode  Ron=FC.Rohm  Lon=0  Vf=0  IC=0  UseSnubber=off  Rs=1e4  Cs=inf  Measurements=off
  FuelFr : Constant  Value=FC.Uf_H2
  Gain1 : Gain  Gain=0.01
  Gain3 : Gain  Gain=0.01
  Model : spsFuelCellModel/Fuel Cell model  SystemSampleTime=-1  LabelModeActiveChoice=Continuous/Detailed  VariantActivationTime=update diagram  Latency=0  AutoFrameSizeCalculation=off
      settings: AttributesFormatString=%<BlockChoice>  SourceProductBaseCode=PS
  PAir : Constant  Value=FC.PAir
  Pfuel : Constant  Value=FC.Pf
  T : Constant  Value=FC.Tnom
  x_H2 : Constant  Value=FC.x*100
  y_O2 : Constant  Value=FC.y*100
  + : PMIOPort  Tag=PMCPort  Side=Right
  - : PMIOPort  Tag=PMCPort  Port=2  Side=Right
  m : Outport  VectorParamsAs1DForOutWhenUnconnected=off
  wires:
  PAir/1 -> Model/8
  Pfuel/1 -> Model/7
  T/1 -> Model/2
  Model/1 -> Controlled Voltage Source1/1
  Current Measurement1/1 -> Model/1
  Model/2 -> m/1
  FuelFr/1 -> Model/3
  x_H2/1 -> Gain1/1
  AirFr/1 -> Model/5
  y_O2/1 -> Gain3/1
  Gain1/1 -> Model/4
  Gain3/1 -> Model/6
  connections:
  Current Measurement1/LConn1 -- Controlled Voltage Source1/RConn1
  Diode1/LConn1 -- Current Measurement1/RConn1
  -/RConn1 -- Controlled Voltage Source1/LConn1
  Diode1/RConn1 -- +/RConn1

== system SIM_PEM_stack/5 PEM stack3/Fuel Cell Stack5 ==
  AirFr : Constant  Value=FC.Uf_O2
  Controlled Voltage Source1 : powerlib/Electrical Sources/Controlled Voltage Source  Initialize=on  Source_Type=AC  Amplitude=0  Phase=0  Frequency=0  Measurements=None
  Current Measurement : powerlib/Measurements/Current Measurement  PhasorSimulation=off  OutputType=Complex  PSBequivalent=0
  Current Measurement1 : powerlib/Measurements/Current Measurement  PhasorSimulation=off  OutputType=Complex  PSBequivalent=0
  Diode1 : powerlib/Power Electronics/Diode  Ron=FC.Rohm  Lon=0  Vf=0  IC=0  UseSnubber=off  Rs=1e4  Cs=inf  Measurements=off
  FuelFr : Constant  Value=FC.Uf_H2
  Gain1 : Gain  Gain=0.01
  Gain3 : Gain  Gain=0.01
  Model : spsFuelCellModel/Fuel Cell model  SystemSampleTime=-1  LabelModeActiveChoice=Continuous/Detailed  VariantActivationTime=update diagram  Latency=0  AutoFrameSizeCalculation=off
      settings: AttributesFormatString=%<BlockChoice>  SourceProductBaseCode=PS
  PAir : Constant  Value=FC.PAir
  Pfuel : Constant  Value=FC.Pf
  T : Constant  Value=FC.Tnom
  x_H2 : Constant  Value=FC.x*100
  y_O2 : Constant  Value=FC.y*100
  + : PMIOPort  Tag=PMCPort  Side=Right
  - : PMIOPort  Tag=PMCPort  Port=2  Side=Right
  m : Outport  VectorParamsAs1DForOutWhenUnconnected=off
  wires:
  PAir/1 -> Model/8
  Pfuel/1 -> Model/7
  T/1 -> Model/2
  Model/1 -> Controlled Voltage Source1/1
  Current Measurement1/1 -> Model/1
  Model/2 -> m/1
  FuelFr/1 -> Model/3
  x_H2/1 -> Gain1/1
  AirFr/1 -> Model/5
  y_O2/1 -> Gain3/1
  Gain1/1 -> Model/4
  Gain3/1 -> Model/6
  connections:
  Current Measurement1/LConn1 -- Controlled Voltage Source1/RConn1
  Diode1/LConn1 -- Current Measurement1/RConn1
  -/RConn1 -- Controlled Voltage Source1/LConn1
  Diode1/RConn1 -- +/RConn1
